simulink model "hinf_test"  (R2015b)
settings: Solver=VariableStepAuto  StartTime=0.0  StopTime=80.0  RelTol=1e-3
values from neighbouring files (symbols this model uses):
  T = sysic    [h_infinito.m]    (also in mu_controller.m)
undefined symbols (not defined in the file or in its folder): Ks_inf, pulsazione
settings Model: Creator=michele  LastModifiedBy=michele

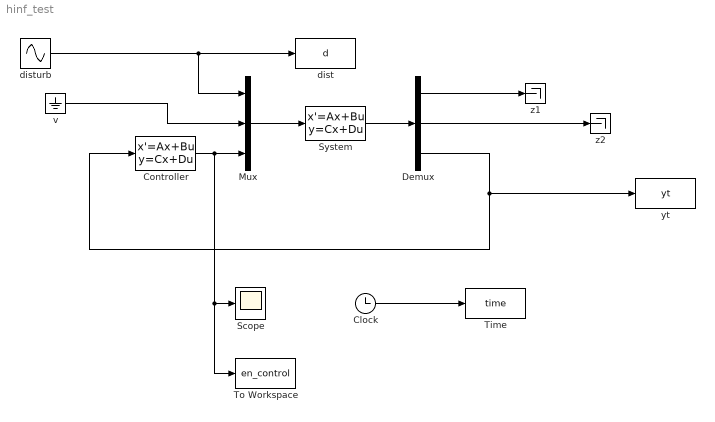
== system hinf_test ==
  Clock : Clock
  Controller : StateSpace  A=Ks_inf.a  B=Ks_inf.b  C=Ks_inf.c  D=Ks_inf.d  X0=0
  Demux : Demux  Outputs=3
  Mux : Mux  Inputs=3
  Scope : Scope
  System : StateSpace  A=T.NominalValue.a  B=T.NominalValue.b  C=T.NominalValue.c  D=T.NominalValue.d  X0=0
  Time : ToWorkspace  VariableName=time  SaveFormat=Timeseries  SampleTime=-1
  To Workspace : ToWorkspace  VariableName=en_control  SaveFormat=Timeseries  SampleTime=-1
  dist : ToWorkspace  VariableName=d  SaveFormat=Timeseries  SampleTime=-1
  disturb : Sin  Frequency=pulsazione  SampleTime=0
  v : Ground
  yt : ToWorkspace  VariableName=yt  SaveFormat=Timeseries  SampleTime=-1
  z1 : Terminator
  z2 : Terminator
  wires:
  Mux/1 -> System/1
  System/1 -> Demux/1
  Demux/3 -> yt/1, Controller/1
  Controller/1 -> To Workspace/1, Scope/1, Mux/3
  Demux/2 -> z2/1
  Demux/1 -> z1/1
  v/1 -> Mux/2
  Clock/1 -> Time/1
  disturb/1 -> Mux/1, dist/1
